simulink model "elevator"  (R2017b)
settings: Solver=FixedStepDiscrete  StartTime=0.0  StopTime=10.0  RelTol=1e-3
libraries: arduinolib x7, simulink x1
settings Model: ExtModeTrigDuration=2  Creator=Albin  LastModifiedBy=Albin
settings RTWCC: BuildConfiguration=Faster Runs

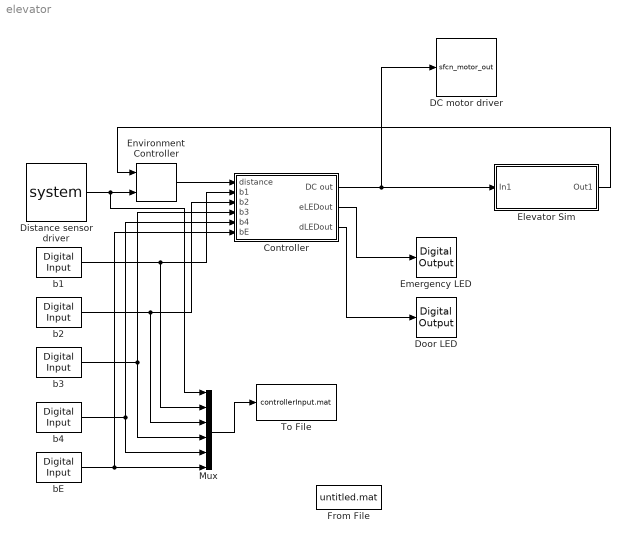
== system elevator ==
  Controller : Subsystem
  DC motor driver : S-Function  InitFcn=try, set_param(gcb,'FunctionName','sfcn_motor_out'), end  FunctionName=sfcn_motor_out  Parameters=uint8(10),uint8(9),uint8(11)  SFunctionModules=sfcn_motor_out_wrapper  SFunctionDeploymentMode=off  EnableBusSupport=off  mask(S-Function Builder){}
      mask help: Simulink:masks:SFunctionBuilder_MD
      mask init:
      | val = [[.9  0.75 0.75 1 1 .9 .9 1]',[1 1 0.75 0.75 .9 .9 1 .9]'];try , sys = get_param(gcb,'SfunBuilderFcnName');if isempty(sys), sys = get_param(gcb,'FunctionName'); end,catch, sys = get_param(gcb,'FunctionName'); end
      settings: CopyFcn=set_param(gcbh,'LinkStatus','none')  PreSaveFcn=try, set_param(gcb,'FunctionName','sfcn_motor_out'), end  OpenFcn=sfunctionwizard(gcbh)
      mask Display: plot(val(:,1),val(:,2)),disp(sys), port_label('input',1,'in')
  Distance sensor driver : S-Function  InitFcn=try, set_param(gcb,'FunctionName','sfcn_sensor_in'), end  Parameters=uint8(2),uint8(3)  SFunctionDeploymentMode=off  EnableBusSupport=off  mask(S-Function Builder){}
      mask help: Simulink:masks:SFunctionBuilder_MD
      mask init: same as elevator/DC motor driver
      settings: CopyFcn=set_param(gcbh,'LinkStatus','none')  PreSaveFcn=try, set_param(gcb,'FunctionName',''), end  OpenFcn=sfunctionwizard(gcbh)
      mask Display: plot(val(:,1),val(:,2)),disp(sys), port_label('input',1,'u0'), port_label('output',1,'y0')
  Door LED : arduinolib/Digital Output  pinNumber=5  blockPlatform=arduino
  Elevator Sim : Subsystem
  Emergency LED : arduinolib/Digital Output  pinNumber=4  blockPlatform=arduino
  Environment Controller : simulink/Signal Routing/Environment Controller
      settings: SourceProductName=Simulink  SourceProductBaseCode=SL
  From File : FromFile  SampleTime=0
  Mux : Mux  Inputs=6
  To File : ToFile  Filename=controllerInput.mat  MatrixName=loggedInput  SaveFormat=Timeseries
  b{1..4} (4 alike) : arduinolib/Digital Input  pinNumber=6  sampleTime=0.1  blockPlatform=arduino
      settings: SourceProductName=Simulink Support Package for Arduino Hardware
  bE : arduinolib/Digital Input  pinNumber=6  sampleTime=0.1  blockPlatform=arduino
      settings: SourceProductName=Simulink Support Package for Arduino Hardware
  wires:
  Environment Controller/1 -> Controller/1(distance)
  Elevator Sim/1(Out1) -> Environment Controller/1
  Distance sensor driver/1 -> Mux/1, Environment Controller/2
  Controller/1(DC out) -> DC motor driver/1, Elevator Sim/1(In1)
  Controller/2(eLEDout) -> Emergency LED/1
  Controller/3(dLEDout) -> Door LED/1
  b1/1 -> Mux/2, Controller/2(b1)
  b2/1 -> Mux/3, Controller/3(b2)
  b3/1 -> Mux/4, Controller/4(b3)
  b4/1 -> Mux/5, Controller/5(b4)
  bE/1 -> Mux/6, Controller/6(bE)
  Mux/1 -> To File/1

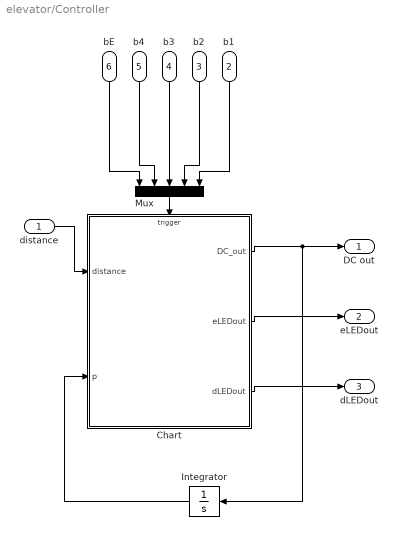
== system elevator/Controller ==
  distance : Inport
  b1 : Inport  Port=2
  b2 : Inport  Port=3
  b3 : Inport  Port=4
  b4 : Inport  Port=5
  bE : Inport  Port=6
  Chart : Stateflow chart  TreatAsAtomicUnit=on
  Integrator : Integrator
  Mux : Mux  Inputs=5
  DC out : Outport
  eLEDout : Outport  Port=2
  dLEDout : Outport  Port=3
  wires:
  distance/1 -> Chart/1(distance)
  Chart/1(DC_out) -> Integrator/1, DC out/1
  Chart/2(eLEDout) -> eLEDout/1
  Chart/3(dLEDout) -> dLEDout/1
  Integrator/1 -> Chart/2(p)
  Mux/1 -> Chart/Trigger
  b1/1 -> Mux/5
  b2/1 -> Mux/4
  b3/1 -> Mux/3
  b4/1 -> Mux/2
  bE/1 -> Mux/1

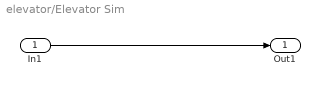
== system elevator/Elevator Sim ==
  In1 : Inport
  Out1 : Outport
  wires:
  In1/1 -> Out1/1

== stateflow chart elevator/Controller/Chart ==
  settings: executeAtInitialization=1
  state Stop
    en: DC_out = 0;
    en: eLEDout = 1;
    ex: eLEDout = 0;
  state Normal
    (history)
    state Position [parallel]
      settings: executionOrder=1
      state Floor
        (history)
        state floor1
          en: currentFloor = 1;
        state floor2
          en: currentFloor = 2;
        state floor3
          en: currentFloor = 3;
        state floor4
          en: currentFloor = 4;
        floor2 -> floor1 [order 1] : [distance < floor1dist + margin && pressed(1)]/{pressed(1)=false;send(STOP)}
        floor1 -> floor2 [order 1] : [distance > floor2dist - margin && pressed(2)]/{pressed(2)=false;send(STOP)}
        floor1 -> floor2 [order 2] : [distance > floor4dist - margin]
        floor2 -> floor1 [order 4] : [distance < floor1dist + margin ]
        floor3 -> floor2 [order 2] : [distance < floor2dist + margin && pressed(2)]/{pressed(2)=false;send(STOP)}
        floor2 -> floor3 [order 2] : [distance > floor3dist - margin && pressed(3)]/{pressed(3)=false;send(STOP)}
        floor2 -> floor3 [order 3] : [distance > floor3dist - margin]
        floor3 -> floor2 [order 4] : [distance < floor2dist + margin]
        floor4 -> floor3 [order 1] : [distance < floor3dist + margin && pressed(3)]/{pressed(3)=false;send(STOP)}
        floor3 -> floor4 [order 1] : [distance > floor4dist - margin && pressed(4)]/{pressed(4)=false;send(STOP)}
        floor3 -> floor4 [order 3] : [distance > floor4dist - margin]
        floor4 -> floor3 [order 2] : [distance < floor2dist + margin ]
      state stopped
        state doorClosed
        state doorOpen
          en: dLEDout = 1;
        doorOpen -> doorClosed : after(5, secs)
      doorClosed -> Floor : START
      Floor -> doorOpen : STOP
    state Set direction [parallel]
      settings: executionOrder=3
    state enqueue [parallel]
      settings: executionOrder=2
    Set direction -> Set direction : [~pressed(1) && ~pressed(2) && ~pressed(3) && ~pressed(4)]/{direction = 0}
    enqueue -> enqueue [order 4] : B4/{pressed(4)=true;}
    enqueue -> enqueue [order 3] : B3/{pressed(3)=true;}
    enqueue -> enqueue [order 2] : B2/{pressed(2)=true;}
    enqueue -> enqueue [order 1] : B1/{pressed(1)=true;}
  state Initialization
  Normal -> Stop : BE
  Stop -> Normal : BE
  Initialization -> floor1
  (default) -> Initialization
  data: distance input; DC_out output; eLEDout output; dLEDout output; p input; pressed local boolean size=5; currentFloor local
  events: B1 input RISING_EDGE_EVENT; B2 input RISING_EDGE_EVENT; B3 input RISING_EDGE_EVENT; B4 input RISING_EDGE_EVENT; BE input RISING_EDGE_EVENT; TODOany local FUNCTION_CALL_EVENT; STOP local FUNCTION_CALL_EVENT; START local FUNCTION_CALL_EVENT; B5 input FUNCTION_CALL_EVENT
